simulink model "ProjectSimulink"  (R2021a)
settings: Solver=ode23  StartTime=60000  StopTime=70000  MaxStep=0.01  RelTol=1e-3
values from neighbouring files (symbols this model uses):
  Cn = Cn_cell*Np    [ProjectMatlab_Final.m]
  diesel_cap_pu = diesel_cap/Psysbase    (= 0.284375)    [ProjectMatlab_Final.m]
  EFF = 0.93    [ProjectMatlab_Final.m]
  H = 5    [ProjectMatlab_Final.m]
  k = 0.5    [ProjectMatlab_Final.m]
  k_bat = 0.5    [ProjectMatlab_Final.m]
  k_PV = 0.5    [ProjectMatlab_Final.m]
  Kii = wi^2*L/udc    (= 0.000555555555556)    [ProjectMatlab_Final.m]
  Kpi = 2*xii*wi*L/udc    (= 7.77777777778e-05)    [ProjectMatlab_Final.m]
  Ksoc = 100*(Irated*0.05)    [ProjectMatlab_Final.m]
  L = 0.005    [ProjectMatlab_Final.m]
  load_0 = 0.5    [ProjectMatlab_Final.m]
  load_0_bat = (load_0 - penetration)*Psysbase/Pgenbase    (= -0.3)    [ProjectMatlab_Final.m]
  load_0_synch = 0    [ProjectMatlab_Final.m]
  OCV_0 = interp1(SOC_LUT,OCV_LUT,SOC_0,'linear','extrap')    [ProjectMatlab_Final.m]
  OCV_LUT = Ns*OCV_LUT_cell'    [ProjectMatlab_Final.m]
  Psysbase = 320    [ProjectMatlab_Final.m]
  R = 0.03    [ProjectMatlab_Final.m]
  R_PV = 0.1    [ProjectMatlab_Final.m]
  Rb = R_cell*Ns/Np    [ProjectMatlab_Final.m]
  Rf = 0.05    [ProjectMatlab_Final.m]
  SOC_0 = 0.7    [ProjectMatlab_Final.m]
  SOC_LUT = [0.0066 0.1004 0.2004 0.3003 0.4002 0.5002 0.6001 0.7000 0.8000 0.8999 0.9998]'    [ProjectMatlab_Final.m]
  storage_p = bat_power_cap/Psysbase    (= 0.3343125)    [ProjectMatlab_Final.m]
  TCH = 0.3    [ProjectMatlab_Final.m]
  TG = 0.2    [ProjectMatlab_Final.m]
  Ub_exp = max(OCV_LUT)    [ProjectMatlab_Final.m]
  Ub_min = min(OCV_LUT)    [ProjectMatlab_Final.m]
  udc = storage_u * 1.5    (= 900)    [ProjectMatlab_Final.m]
  wbase = 2*pi*50    (= 314.159265359)    [ProjectMatlab_Final.m]
libraries: simulink x6
settings Model: Creator=bendiksherbold  LastModifiedBy=bendiksherbold
settings SolverCC: ZeroCrossAlgorithm=Adaptive
settings DataIOCC: ExternalInput=pv_data,timeseries_load  LoadExternalInput=on
settings DebuggingCC: IgnoredZcDiagnostic=none

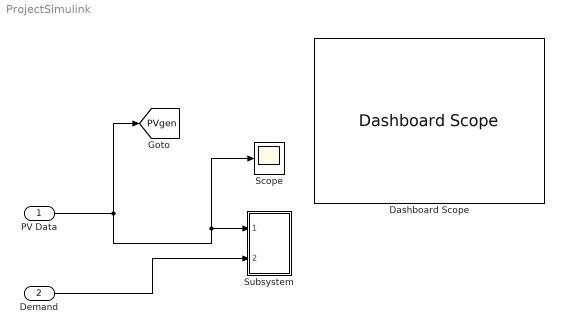
== system ProjectSimulink ==
  PV Data : Inport
  Demand : Inport  Port=2
  Dashboard Scope : DashboardScope
  Scope : Scope
  Subsystem : Subsystem
  tag scope: PVgen=global
  wires:
  PV Data/1 -> Scope/1, Subsystem/1(Renewables Input), [PVgen]
  Demand/1 -> Subsystem/2(Demand)

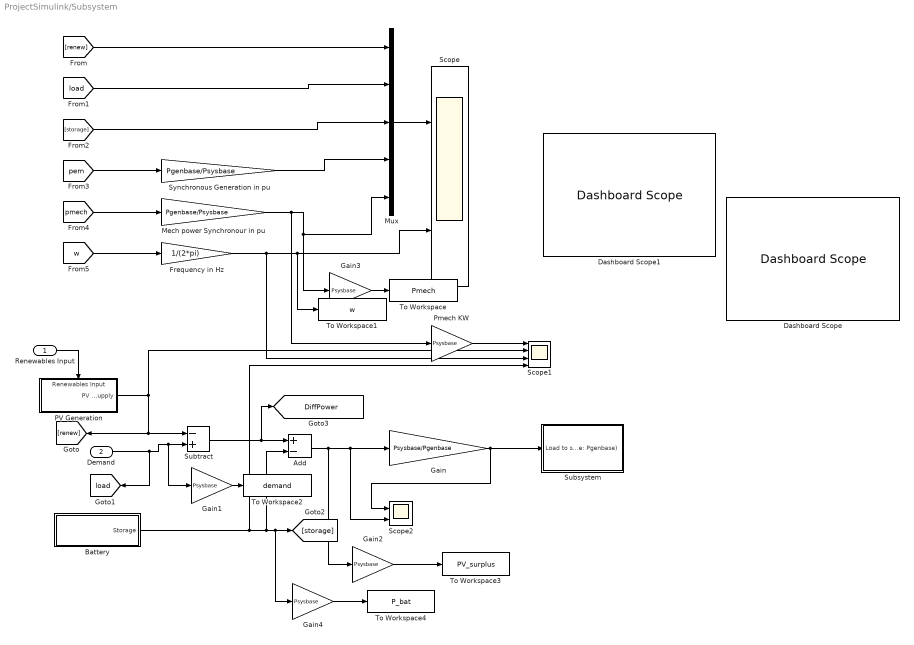
== system ProjectSimulink/Subsystem ==
  Renewables Input : Inport
  Demand : Inport  Port=2
  Add : Sum  Inputs=+-
  Battery : Subsystem
  Dashboard Scope : DashboardScope
  Dashboard Scope1 : DashboardScope
  Frequency in Hz : Gain  Gain=1/(2*pi)
  Gain : Gain  Gain=Psysbase/Pgenbase
  Gain{1..4} (4 alike) : Gain  Gain=Psysbase
  Mech power Synchronour in pu : Gain  Gain=Pgenbase/Psysbase
  Mux : Mux  Inputs=5
  PV Generation : Subsystem
      settings: PortSchema="{\"entries\":[{\"content\":{\"sides\":[{\"content\":{\"connectorIds\":[]},\"type\":\"ConnectorPlacement.EquallySpacedRectSide\",\"uuid\":\"0eea5417-339e-48e3-be8a-7ac1e3b13c5e\"},{\"content\":{\"connectorIds\":[\"Out1\"],\"side\":\"RIGHT\"},\"type\":\"ConnectorPlacement.EquallySpacedRectSide\",\"uuid\":\"a12bbc12-1de9-45f8-93a0-544242284c74\"},{\"content\":{\"connectorIds\":[\"In1\"],\"side\":\"TOP\"},\"type\":\"ConnectorPlacement.EquallySpacedRectSide\",\"uuid\":\"cdfd9bc5-7ff1-4687-a49b-7b50cbbba0d4\"}]},\"type\":\"ConnectorPlacement.EquallySpacedConnector\",\"uuid\":\"d3b80c90-fca6-417c-b380-4dfc861acc4c\"}],\"packageUris\":[\"http://schema.mathworks.com/mf0/Connector/R2020b\"],\"version\":\"1.0\"}"
  Pmech KW : Gain  Gain=Psysbase
  Scope : Scope  NumInputPorts=2
  Scope1 : Scope  NumInputPorts=4
  Scope2 : Scope  NumInputPorts=2
  Subsystem : Subsystem
  Subtract : Sum  Inputs=-+
  Synchronous Generation in pu : Gain  Gain=Pgenbase/Psysbase
  To Workspace : ToWorkspace  VariableName=Pmech  SaveFormat=Timeseries  SampleTime=-1
  To Workspace1 : ToWorkspace  VariableName=w  SaveFormat=Timeseries  SampleTime=-1
  To Workspace2 : ToWorkspace  VariableName=demand  SaveFormat=Timeseries  SampleTime=-1
  To Workspace3 : ToWorkspace  VariableName=PV_surplus  SaveFormat=Timeseries  SampleTime=-1
  To Workspace4 : ToWorkspace  VariableName=P_bat  SaveFormat=Timeseries  SampleTime=-1
  tag scope: DiffPower=global, load=global
  wires:
  [renew] -> Mux/1
  [load] -> Mux/2
  [storage] -> Mux/3
  [pem] -> Synchronous Generation in pu/1
  Synchronous Generation in pu/1 -> Mux/4
  [pmech] -> Mech power Synchronour in pu/1
  [w] -> Frequency in Hz/1
  Mux/1 -> Scope/1
  Frequency in Hz/1 -> Scope1/3, To Workspace1/1, Scope/2
  Gain/1 -> Subsystem/1(Load to synch generator (pu base: Pgenbase)), Scope2/1
  Subtract/1 -> Add/1, [DiffPower]
  Battery/1(Storage) -> Scope1/4, Add/2, Gain4/1, [storage]
  Add/1 -> Gain2/1, Scope2/2, Gain/1
  PV Generation/1(PV Power supply) -> [renew], Subtract/1, Scope1/2
  Renewables Input/1 -> PV Generation/1(Renewables Input)
  Demand/1 -> [load], Gain1/1, Subtract/2
  Gain1/1 -> To Workspace2/1
  Gain2/1 -> To Workspace3/1
  Gain3/1 -> To Workspace/1
  Mech power Synchronour in pu/1 -> Pmech KW/1, Mux/5, Gain3/1
  Pmech KW/1 -> Scope1/1
  Gain4/1 -> To Workspace4/1

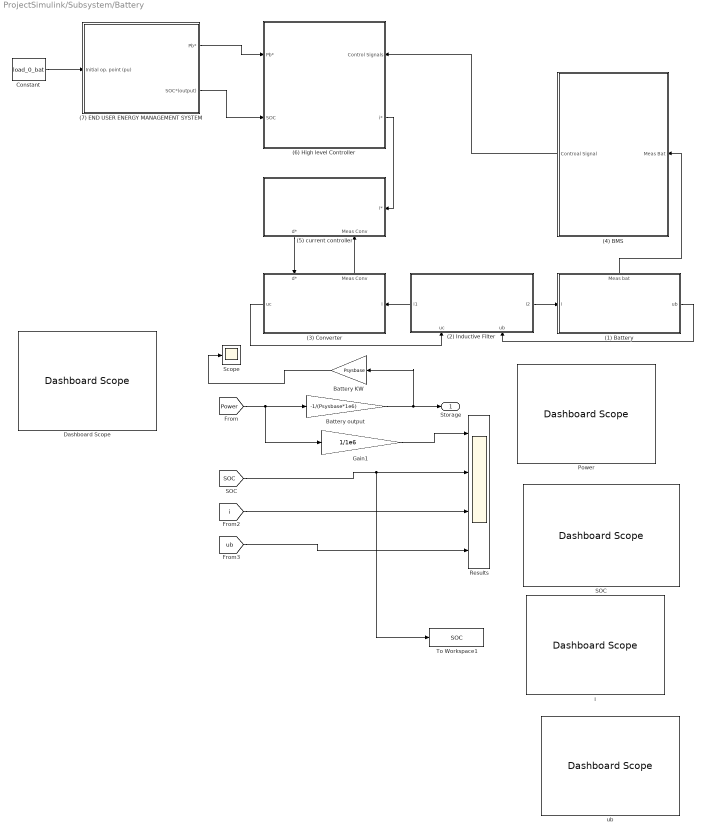
== system ProjectSimulink/Subsystem/Battery ==
  " SOC" : DashboardScope
  (1) Battery : Subsystem
      settings: PortSchema="{\"entries\":[{\"content\":{\"sides\":[{\"content\":{\"connectorIds\":[\"In1\"]},\"type\":\"ConnectorPlacement.EquallySpacedRectSide\",\"uuid\":\"e34c45c3-0268-41b7-a456-a7ff7a17db6e\"},{\"content\":{\"connectorIds\":[\"Out1\"],\"side\":\"RIGHT\"},\"type\":\"ConnectorPlacement.EquallySpacedRectSide\",\"uuid\":\"7704b9d9-7556-456b-9f5a-c4d56f80ae30\"},{\"content\":{\"connectorIds\":[\"Out2\"],\"side\":\"TOP\"},\"type\":\"ConnectorPlacement.EquallySpacedRectSide\",\"uuid\":\"0449123b-420b-4c01-93d9-a7aad71b96da\"}]},\"type\":\"ConnectorPlacement.EquallySpacedConnector\",\"uuid\":\"13f32f51-f15f-4766-88e8-e2ed957cd412\"}],\"packageUris\":[\"http://schema.mathworks.com/mf0/Connector/R2020b\"],\"version\":\"1.0\"}"
  (2) Inductive Filter : Subsystem
      settings: PortSchema="{\"entries\":[{\"content\":{\"sides\":[{\"content\":{\"connectorIds\":[\"Out2\"]},\"type\":\"ConnectorPlacement.EquallySpacedRectSide\",\"uuid\":\"c9490074-2b7b-4447-a33c-a9379d322631\"},{\"content\":{\"connectorIds\":[\"Out1\"],\"side\":\"RIGHT\"},\"type\":\"ConnectorPlacement.EquallySpacedRectSide\",\"uuid\":\"2ec79e2c-d8dd-4257-943e-016b77f5a984\"},{\"content\":{\"connectorIds\":[],\"side\":\"TOP\"},\"type\":\"ConnectorPlacement.EquallySpacedRectSide\",\"uuid\":\"d6c4e837-3256-4e0a-b933-06ad8d5ab609\"},{\"content\":{\"connectorIds\":[\"In1\",\"In2\"],\"side\":\"BOTTOM\"},\"type\":\"ConnectorPlacement.EquallySpacedRectSide\",\"uuid\":\"4075f384-4c82-404c-bba4-24b3ea83b751\"}]},\"type\":\"ConnectorPlacement.EquallySpacedConnector\",\"uuid\":\"d50deaef-6ab5-4075-8ac8-83e9d6338d4a\"}],\"packageUris\":[\"http://schema.mathworks.com/mf0/Connector/R2020b\"],\"version\":\"1.0\"}"
  (3) Converter : Subsystem
      settings: PortSchema="{\"entries\":[{\"content\":{\"sides\":[{\"content\":{\"connectorIds\":[\"Out2\"]},\"type\":\"ConnectorPlacement.EquallySpacedRectSide\",\"uuid\":\"c9490074-2b7b-4447-a33c-a9379d322631\"},{\"content\":{\"connectorIds\":[\"In2\"],\"side\":\"RIGHT\"},\"type\":\"ConnectorPlacement.EquallySpacedRectSide\",\"uuid\":\"2ec79e2c-d8dd-4257-943e-016b77f5a984\"},{\"content\":{\"connectorIds\":[\"In1\",\"Out1\"],\"side\":\"TOP\"},\"type\":\"ConnectorPlacement.EquallySpacedRectSide\",\"uuid\":\"d6c4e837-3256-4e0a-b933-06ad8d5ab609\"}]},\"type\":\"ConnectorPlacement.EquallySpacedConnector\",\"uuid\":\"d50deaef-6ab5-4075-8ac8-83e9d6338d4a\"}],\"packageUris\":[\"http://schema.mathworks.com/mf0/Connector/R2020b\"],\"version\":\"1.0\"}"
  (4) BMS : Subsystem
      settings: PortSchema="{\"entries\":[{\"content\":{\"sides\":[{\"content\":{\"connectorIds\":[\"Out1\"]},\"type\":\"ConnectorPlacement.EquallySpacedRectSide\",\"uuid\":\"7ad5997f-ae27-4a98-8ab9-418effdbae5c\"},{\"content\":{\"connectorIds\":[\"In1\"],\"side\":\"RIGHT\"},\"type\":\"ConnectorPlacement.EquallySpacedRectSide\",\"uuid\":\"c56e7a01-525e-484f-a434-88ecf8a546e8\"},{\"content\":{\"connectorIds\":[],\"side\":\"TOP\"},\"type\":\"ConnectorPlacement.EquallySpacedRectSide\",\"uuid\":\"617b0b0b-0700-4f1b-a6c2-75a7b65ee563\"},{\"content\":{\"connectorIds\":[],\"side\":\"BOTTOM\"},\"type\":\"ConnectorPlacement.EquallySpacedRectSide\",\"uuid\":\"8f108a49-84c7-4e3f-a676-05e2ecd3a647\"}]},\"type\":\"ConnectorPlacement.EquallySpacedConnector\",\"uuid\":\"a459534c-8992-4e34-9193-d09d3abfd6a6\"}],\"packageUris\":[\"http://schema.mathworks.com/mf0/Connector/R2020b\"],\"version\":\"1.0\"}"
  (5) current controller : Subsystem
      settings: PortSchema="{\"entries\":[{\"content\":{\"sides\":[{\"content\":{\"connectorIds\":[]},\"type\":\"ConnectorPlacement.EquallySpacedRectSide\",\"uuid\":\"2d354075-c17d-4344-a815-85536605997e\"},{\"content\":{\"connectorIds\":[\"In2\"],\"side\":\"RIGHT\"},\"type\":\"ConnectorPlacement.EquallySpacedRectSide\",\"uuid\":\"9e91ce6a-f1ef-4336-bc5a-278a409c018d\"},{\"content\":{\"connectorIds\":[],\"side\":\"TOP\"},\"type\":\"ConnectorPlacement.EquallySpacedRectSide\",\"uuid\":\"a4716af3-f2b8-45e2-a3c3-6e76ca82c58b\"},{\"content\":{\"connectorIds\":[\"Out1\",\"In1\"],\"side\":\"BOTTOM\"},\"type\":\"ConnectorPlacement.EquallySpacedRectSide\",\"uuid\":\"8f9d6488-9f86-4c0c-8bcc-8928f445b617\"}]},\"type\":\"ConnectorPlacement.EquallySpacedConnector\",\"uuid\":\"f4ac1926-eca6-4ae4-a6e1-7b825295d917\"}],\"packageUris\":[\"http://schema.mathworks.com/mf0/Connector/R2020b\"],\"version\":\"1.0\"}"
  (6) High level Controller : Subsystem
      settings: PortSchema="{\"entries\":[{\"content\":{\"sides\":[{\"content\":{\"connectorIds\":[\"In1\",\"In2\"]},\"type\":\"ConnectorPlacement.EquallySpacedRectSide\",\"uuid\":\"f1980330-cce1-4eae-bd21-bb2edf6a6354\"},{\"content\":{\"connectorIds\":[\"In3\",\"Out1\"],\"side\":\"RIGHT\"},\"type\":\"ConnectorPlacement.EquallySpacedRectSide\",\"uuid\":\"5b150bd5-b030-427f-a8ee-89c6d0847365\"},{\"content\":{\"connectorIds\":[],\"side\":\"TOP\"},\"type\":\"ConnectorPlacement.EquallySpacedRectSide\",\"uuid\":\"ea0f71d8-017f-4572-8166-56d940581349\"}]},\"type\":\"ConnectorPlacement.EquallySpacedConnector\",\"uuid\":\"37bf4f98-7efc-4bdf-9457-78864a4c59b2\"}],\"packageUris\":[\"http://schema.mathworks.com/mf0/Connector/R2020b\"],\"version\":\"1.0\"}"
  (7) END USER ENERGY MANAGEMENT SYSTEM : Subsystem
  Battery KW : Gain  Gain=Psysbase
  Battery output : Gain  Gain=-1/(Psysbase*1e6)
  Constant : Constant  Value=load_0_bat
  Dashboard Scope : DashboardScope
  Gain1 : Gain  Gain=1/1e6
  Power : DashboardScope
  Results : Scope  NumInputPorts=4
  Scope : Scope
  To Workspace1 : ToWorkspace  VariableName=SOC  SaveFormat=Timeseries  SampleTime=-1
      settings: Save2DSignal=2-D array (concatenate along first dimension)
  i : DashboardScope
  ub : DashboardScope
  Storage : Outport
  wires:
  (1) Battery/1(ub) -> (2) Inductive Filter/2(ub)
  (2) Inductive Filter/1(i2) -> (1) Battery/1(i)
  (3) Converter/2(uc) -> (2) Inductive Filter/1(uc)
  (2) Inductive Filter/2(i1) -> (3) Converter/2(i)
  (1) Battery/2(Meas bat) -> (4) BMS/1(Meas Bat)
  (5) current controller/1(d*) -> (3) Converter/1(d*)
  (3) Converter/1(Meas Conv) -> (5) current controller/1(Meas Conv)
  [Power] -> Gain1/1, Battery output/1
  Battery output/1 -> Battery KW/1, Storage/1
  [ub] -> Results/4
  [i] -> Results/3
  [SOC] -> To Workspace1/1, Results/2
  Gain1/1 -> Results/1
  (7) END USER ENERGY MANAGEMENT SYSTEM/1(Pb*) -> (6) High level Controller/1(Pb*)
  (7) END USER ENERGY MANAGEMENT SYSTEM/2(SOC*(output)) -> (6) High level Controller/2(SOC)
  (4) BMS/1(Controal Signal) -> (6) High level Controller/3(Control Signals)
  (6) High level Controller/1(i*) -> (5) current controller/2(i*)
  Constant/1 -> (7) END USER ENERGY MANAGEMENT SYSTEM/1(Initial op. point (pu))
  Battery KW/1 -> Scope/1

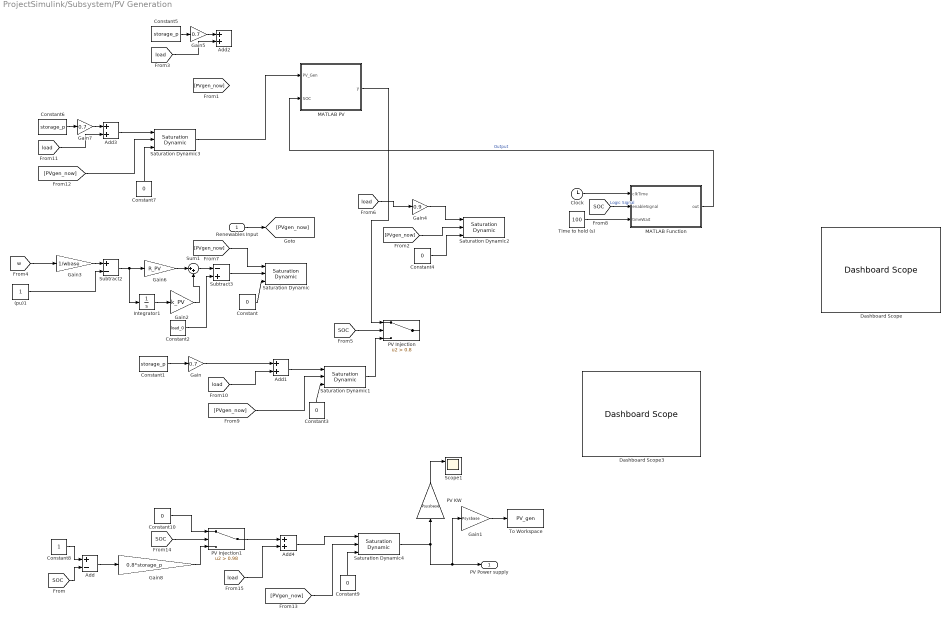
== system ProjectSimulink/Subsystem/PV Generation ==
  Renewables Input : Inport
  (pu)1 : Constant
  Add : Sum  Inputs=+-
  Add{1..4} (4 alike) : Sum
  Clock : Clock
  Constant{,3..4,7,9..10} (6 alike) : Constant  Value=0
  Constant1 : Constant  Value=storage_p
  Constant2 : Constant  Value=load_0
  Constant5 : Constant  Value=storage_p
  Constant6 : Constant  Value=storage_p
  Constant8 : Constant
  Dashboard Scope : DashboardScope
  Dashboard Scope3 : DashboardScope
  Gain : Gain  Gain=0.7
  Gain1 : Gain  Gain=Psysbase
  Gain2 : Gain  Gain=k_PV
  Gain3 : Gain  Gain=1/wbase
  Gain4 : Gain  Gain=0.9
  Gain5 : Gain  Gain=0.7
  Gain6 : Gain  Gain=R_PV
  Gain7 : Gain  Gain=0.7
  Gain8 : Gain  Gain=0.8*storage_p
  Integrator1 : Integrator
  MATLAB Function : MATLAB Function  TreatAsAtomicUnit=on
  MATLAB PV : MATLAB Function  TreatAsAtomicUnit=on
  PV Injection : Switch  Criteria=u2 > Threshold  Threshold=0.8
  PV Injection1 : Switch  Criteria=u2 > Threshold  Threshold=0.98
  PV KW : Gain  Gain=Psysbase
  Saturation Dynamic{,1..4} (5 alike) : simulink/Discontinuities/Saturation Dynamic  OutMin=[]  OutMax=[]  OutDataTypeStr=Inherit: Same as second input  OutDataType=fixdt(1, 16)  OutScaling=2^-10  DoSatur=off
  Scope1 : Scope  NumInputPorts=2
  Subtract2 : Sum  Inputs=+-
  Subtract3 : Sum  Inputs=-+
  Sum1 : Sum  Inputs=|++
  Time to hold (s) : Constant  Value=100
  To Workspace : ToWorkspace  VariableName=PV_gen  SaveFormat=Timeseries  SampleTime=-1
  PV Power supply : Outport
  wires:
  Constant/1 -> Saturation Dynamic/3
  Constant2/1 -> Subtract3/2
  Gain3/1 -> Subtract2/1
  (pu)1/1 -> Subtract2/2
  Subtract2/1 -> Integrator1/1, Gain6/1
  Gain2/1 -> Sum1/2
  Gain6/1 -> Sum1/1
  [w] -> Gain3/1
  Sum1/1 -> Subtract3/1
  Integrator1/1 -> Gain2/1
  Subtract3/1 -> Saturation Dynamic/2
  Renewables Input/1 -> [PVgen_now]
  [PVgen_now] -> Saturation Dynamic/1
  Saturation Dynamic1/1 -> PV Injection/3
  Constant3/1 -> Saturation Dynamic1/3
  Constant1/1 -> Gain/1
  [load] -> Add1/2
  Add1/1 -> Saturation Dynamic1/1
  [PVgen_now] -> Saturation Dynamic1/2
  Gain1/1 -> To Workspace/1
  PV KW/1 -> Scope1/1
  [PVgen_now] -> Saturation Dynamic2/2
  Constant4/1 -> Saturation Dynamic2/3
  Gain/1 -> Add1/1
  [load] -> Gain4/1
  Gain4/1 -> Saturation Dynamic2/1
  [SOC] -> MATLAB Function/2(enableSignal)  "Logic Signal"
  Time to hold (s)/1 -> MATLAB Function/3(timeWait)
  Clock/1 -> MATLAB Function/1(clkTime)
  [SOC] -> PV Injection/2
  MATLAB Function/1(out) -> MATLAB PV/2(SOC)  "Output"
  MATLAB PV/1(y) -> PV Injection/1
  Gain5/1 -> Add2/1
  Constant5/1 -> Gain5/1
  [load] -> Add2/2
  Gain7/1 -> Add3/1
  [PVgen_now] -> Saturation Dynamic3/2
  Constant6/1 -> Gain7/1
  Constant7/1 -> Saturation Dynamic3/3
  [load] -> Add3/2
  Add3/1 -> Saturation Dynamic3/1
  Saturation Dynamic3/1 -> MATLAB PV/1(PV_Gen)
  Constant8/1 -> Add/1
  [SOC] -> Add/2
  Add/1 -> Gain8/1
  [PVgen_now] -> Saturation Dynamic4/2
  Constant9/1 -> Saturation Dynamic4/3
  [SOC] -> PV Injection1/2
  Constant10/1 -> PV Injection1/1
  [load] -> Add4/2
  Add4/1 -> Saturation Dynamic4/1
  Gain8/1 -> PV Injection1/3
  PV Injection1/1 -> Add4/1
  Saturation Dynamic4/1 -> PV KW/1, Gain1/1, PV Power supply/1

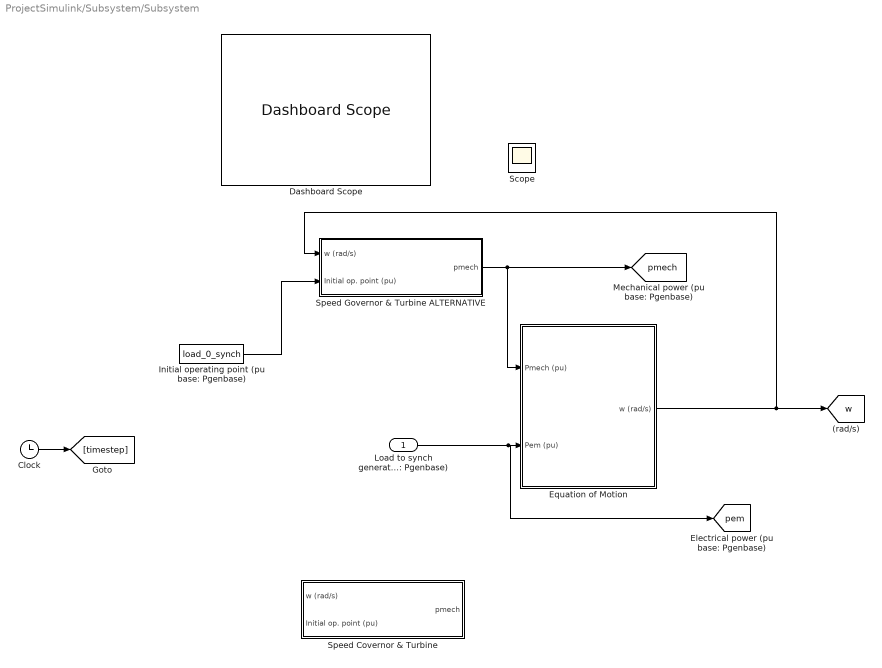
== system ProjectSimulink/Subsystem/Subsystem ==
  Load to synch generator (pu base: Pgenbase) : Inport
  Clock : Clock
  Dashboard Scope : DashboardScope
  Equation of Motion : Subsystem
  Initial operating point (pu base: Pgenbase) : Constant  Value=load_0_synch
  Scope : Scope
  Speed Covernor & Turbine : Subsystem
  Speed Governor & Turbine ALTERNATIVE : Subsystem
  tag scope: pem=global, pmech=global, w=global
  wires:
  Load to synch generator (pu base: Pgenbase)/1 -> [pem], Equation of Motion/2(Pem (pu))
  Equation of Motion/1(w (rad/s)) -> Speed Governor & Turbine ALTERNATIVE/1(w (rad/s)), [w]
  Clock/1 -> [timestep]
  Speed Governor & Turbine ALTERNATIVE/1(pmech) -> Equation of Motion/1(Pmech (pu)), [pmech]
  Initial operating point (pu base: Pgenbase)/1 -> Speed Governor & Turbine ALTERNATIVE/2(Initial op. point (pu))

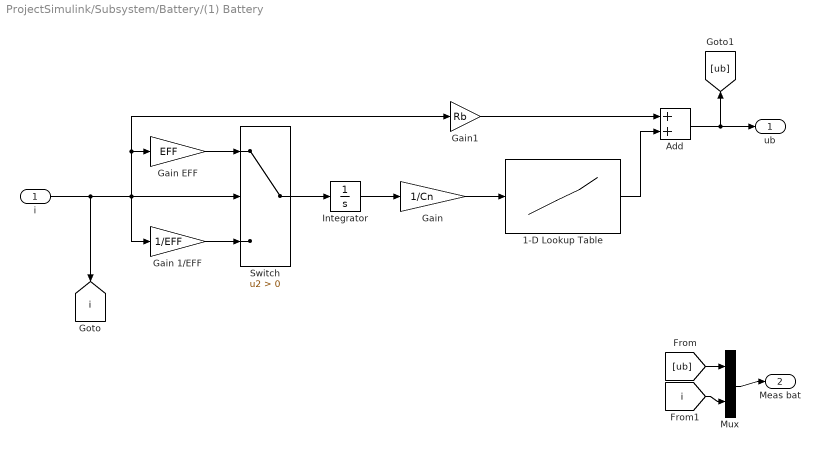
== system ProjectSimulink/Subsystem/Battery/(1) Battery ==
  i : Inport
  1-D Lookup Table : Lookup_n-D  NumberOfTableDimensions=1  BreakpointsForDimension1=SOC_LUT  Table=OCV_LUT  InternalRulePriority=Speed  RndMeth=Simplest  InputSameDT=on
  Add : Sum
  Gain : Gain  Gain=1/Cn
  Gain 1/EFF : Gain  Gain=1/EFF
  Gain EFF : Gain  Gain=EFF
  Gain1 : Gain  Gain=Rb
  Integrator : Integrator  InitialCondition=SOC_0*Cn
  Mux : Mux  Inputs=2
  Switch : Switch  Criteria=u2 > Threshold
  ub : Outport
  Meas bat : Outport  Port=2
  tag scope: i=global
  wires:
  i/1 -> [i], Gain 1/EFF/1, Gain1/1, Gain EFF/1, Switch/2
  Switch/1 -> Integrator/1
  Integrator/1 -> Gain/1
  Gain/1 -> 1-D Lookup Table/1
  Add/1 -> [ub], ub/1
  Gain EFF/1 -> Switch/1
  Gain 1/EFF/1 -> Switch/3
  Gain1/1 -> Add/1
  1-D Lookup Table/1 -> Add/2
  [i] -> Mux/2
  [ub] -> Mux/1
  Mux/1 -> Meas bat/1

== system ProjectSimulink/Subsystem/Battery/(2) Inductive Filter ==
  uc : Inport
  ub : Inport  Port=2
  Add : Sum  Inputs=+-
  Gain : Gain  Gain=1/L
  Integrator : Integrator
  i2 : Outport
  i1 : Outport  Port=2
  wires:
  uc/1 -> Add/1
  ub/1 -> Add/2
  Add/1 -> Gain/1
  Gain/1 -> Integrator/1
  Integrator/1 -> i2/1, i1/1

== system ProjectSimulink/Subsystem/Battery/(3) Converter ==
  d* : Inport
  i : Inport  Port=2
  Gain : Gain  Gain=udc
  Product : Product
  Meas Conv : Outport
  uc : Outport  Port=2
  tag scope: Power=global
  wires:
  d*/1 -> Gain/1
  Gain/1 -> Product/1, uc/1
  i/1 -> Product/2, Meas Conv/1
  Product/1 -> [Power]

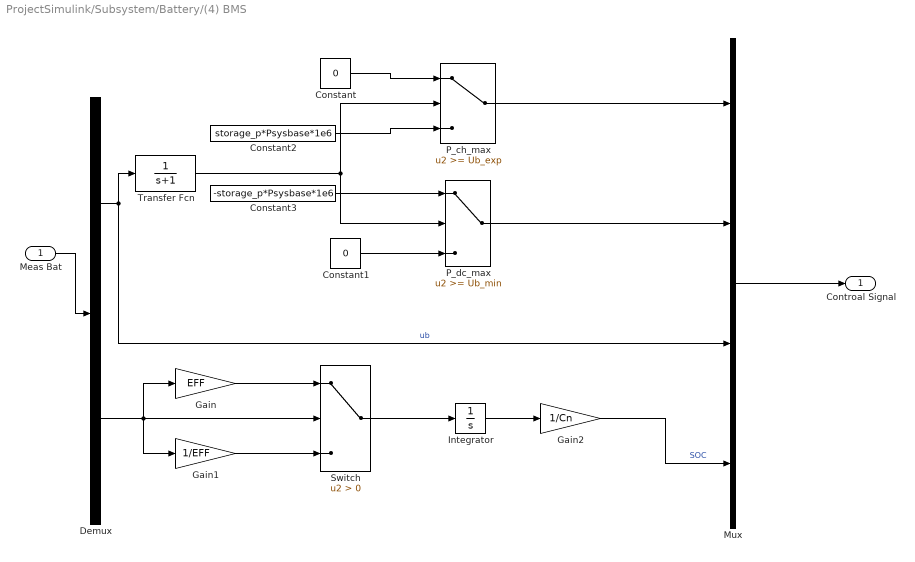
== system ProjectSimulink/Subsystem/Battery/(4) BMS ==
  Meas Bat : Inport
  Constant : Constant  Value=0
  Constant1 : Constant  Value=0
  Constant2 : Constant  Value=storage_p*Psysbase*1e6
  Constant3 : Constant  Value=-storage_p*Psysbase*1e6
  Demux : Demux  Outputs=2
  Gain : Gain  Gain=EFF
  Gain1 : Gain  Gain=1/EFF
  Gain2 : Gain  Gain=1/Cn
  Integrator : Integrator  InitialCondition=SOC_0*Cn
  Mux : Mux
  P_ch_max : Switch  Threshold=Ub_exp  ZeroCross=off
  P_dc_max : Switch  Threshold=Ub_min  ZeroCross=off
  Switch : Switch  Criteria=u2 > Threshold
  Transfer Fcn : TransferFcn  Denominator=[1 1]
  Controal Signal : Outport
  wires:
  Meas Bat/1 -> Demux/1
  Demux/1 -> Transfer Fcn/1, Mux/3  "ub"
  Transfer Fcn/1 -> P_ch_max/2, P_dc_max/2
  Constant/1 -> P_ch_max/1
  Constant1/1 -> P_dc_max/3
  Constant2/1 -> P_ch_max/3
  Constant3/1 -> P_dc_max/1
  Demux/2 -> Gain1/1, Gain/1, Switch/2
  Gain1/1 -> Switch/3
  Gain/1 -> Switch/1
  Switch/1 -> Integrator/1
  Integrator/1 -> Gain2/1
  Gain2/1 -> Mux/4  "SOC"
  P_dc_max/1 -> Mux/2
  P_ch_max/1 -> Mux/1
  Mux/1 -> Controal Signal/1

== system ProjectSimulink/Subsystem/Battery/(5) current controller ==
  Meas Conv : Inport
  i* : Inport  Port=2
  Add : Sum  Inputs=+-
  PI : Subsystem
  d* : Outport
  wires:
  i*/1 -> Add/1
  Meas Conv/1 -> Add/2
  Add/1 -> PI/1(ln)
  PI/1(d*) -> d*/1

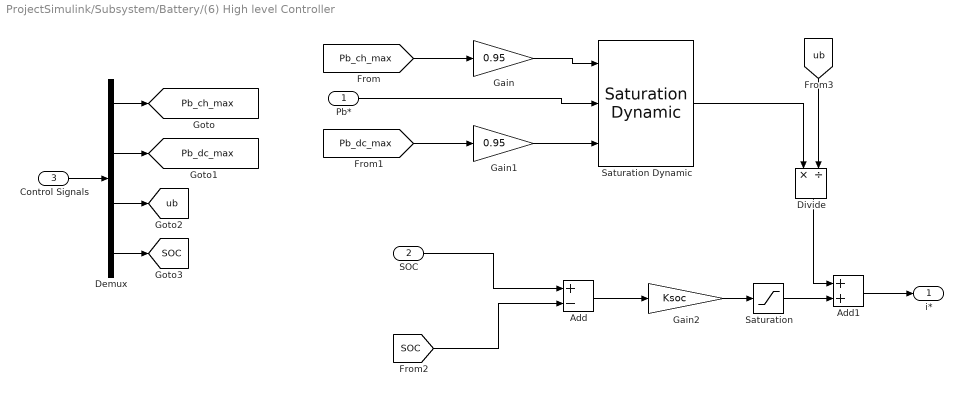
== system ProjectSimulink/Subsystem/Battery/(6) High level Controller ==
  Pb* : Inport
  SOC : Inport  Port=2
  Control Signals : Inport  Port=3
  Add : Sum  Inputs=+-
  Add1 : Sum
  Demux : Demux
  Divide : Product  Inputs=*/
  Gain : Gain  Gain=0.95
  Gain1 : Gain  Gain=0.95
  Gain2 : Gain  Gain=Ksoc
  Saturation : Saturate
  Saturation Dynamic : simulink/Discontinuities/Saturation Dynamic  OutMin=[]  OutMax=[]  OutDataTypeStr=Inherit: Same as second input  OutDataType=fixdt(1, 16)  OutScaling=2^-10  DoSatur=off
  i* : Outport
  tag scope: Pb_ch_max=global, Pb_dc_max=global, SOC=global, ub=global
  wires:
  [Pb_ch_max] -> Gain/1
  [Pb_dc_max] -> Gain1/1
  Pb*/1 -> Saturation Dynamic/2
  Gain/1 -> Saturation Dynamic/1
  Gain1/1 -> Saturation Dynamic/3
  SOC/1 -> Add/1
  [SOC] -> Add/2
  Add/1 -> Gain2/1
  Gain2/1 -> Saturation/1
  Saturation/1 -> Add1/2
  Saturation Dynamic/1 -> Divide/1
  [ub] -> Divide/2
  Divide/1 -> Add1/1
  Add1/1 -> i*/1
  Control Signals/1 -> Demux/1
  Demux/1 -> [Pb_ch_max]
  Demux/2 -> [Pb_dc_max]
  Demux/3 -> [ub]
  Demux/4 -> [SOC]

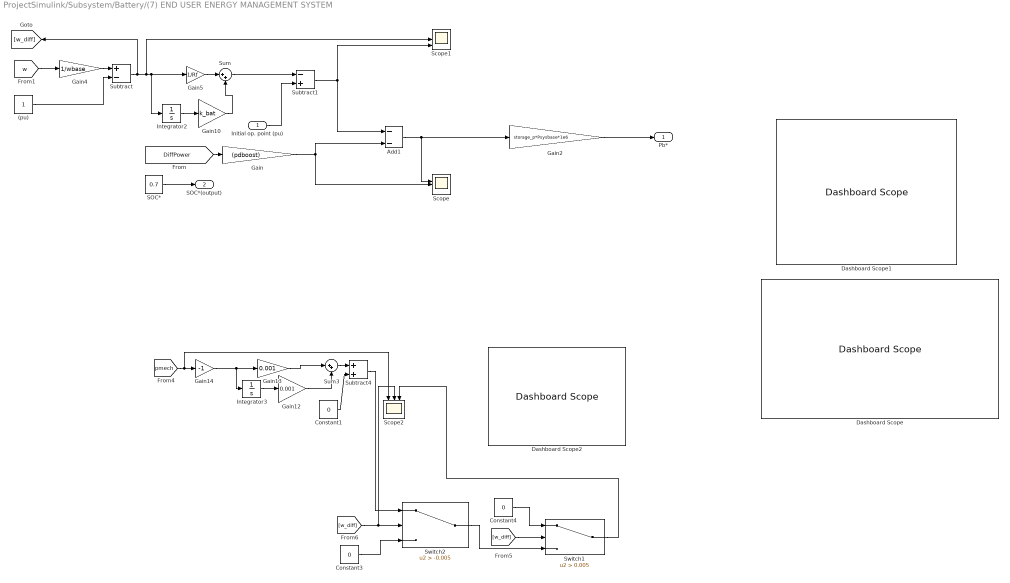
== system ProjectSimulink/Subsystem/Battery/(7) END USER ENERGY MANAGEMENT SYSTEM ==
  Initial op. point (pu) : Inport
  (pu) : Constant
  Add1 : Sum  Inputs=--
  Constant1 : Constant  Value=0
  Constant3 : Constant  Value=0
  Constant4 : Constant  Value=0
  Dashboard Scope : DashboardScope
  Dashboard Scope1 : DashboardScope
  Dashboard Scope2 : DashboardScope
  Gain : Gain  Gain=(pdboost)
  Gain10 : Gain  Gain=k_bat
  Gain12 : Gain  Gain=0.001
  Gain13 : Gain  Gain=0.001
  Gain14 : Gain  Gain=-1
  Gain2 : Gain  Gain=storage_p*Psysbase*1e6
  Gain4 : Gain  Gain=1/wbase
  Gain5 : Gain  Gain=1/Rf
  Integrator2 : Integrator
  Integrator3 : Integrator
  SOC* : Constant  Value=0.7
  Scope : Scope  NumInputPorts=5
  Scope1 : Scope  NumInputPorts=3
  Scope2 : Scope  NumInputPorts=3
  Subtract : Sum  Inputs=+-
  Subtract1 : Sum  Inputs=-+
  Subtract4 : Sum
  Sum : Sum  Inputs=|++
  Sum3 : Sum  Inputs=|++
  Switch1 : Switch  Criteria=u2 > Threshold  Threshold=0.005
  Switch2 : Switch  Criteria=u2 > Threshold  Threshold=-0.005
  Pb* : Outport
  SOC*(output) : Outport  Port=2
  wires:
  [DiffPower] -> Gain/1
  Gain2/1 -> Pb*/1
  SOC*/1 -> SOC*(output)/1
  Gain/1 -> Scope/3, Add1/2
  Gain4/1 -> Subtract/1
  Gain5/1 -> Sum/1
  (pu)/1 -> Subtract/2
  Subtract/1 -> [w_diff], Scope1/2, Integrator2/1, Gain5/1
  Initial op. point (pu)/1 -> Subtract1/2
  Gain10/1 -> Sum/2
  Integrator2/1 -> Gain10/1
  [w] -> Gain4/1
  Sum/1 -> Subtract1/1
  Subtract1/1 -> Scope1/3, Add1/1
  [pmech] -> Scope2/1, Gain14/1
  Integrator3/1 -> Gain12/1
  Gain13/1 -> Sum3/1
  Gain12/1 -> Sum3/2
  Gain14/1 -> Integrator3/1, Gain13/1
  Sum3/1 -> Subtract4/1
  Constant1/1 -> Subtract4/2
  Constant3/1 -> Switch2/3
  [w_diff] -> Switch1/2
  [w_diff] -> Scope2/2, Switch2/2
  Subtract4/1 -> Switch2/1
  Switch1/1 -> Scope2/3
  Constant4/1 -> Switch1/1
  Switch2/1 -> Switch1/3
  Add1/1 -> Gain2/1, Scope/2

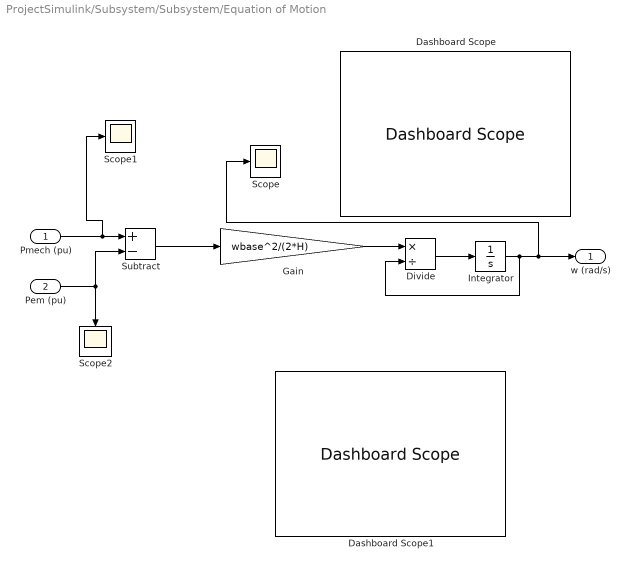
== system ProjectSimulink/Subsystem/Subsystem/Equation of Motion ==
  Pmech (pu) : Inport
  Pem (pu) : Inport  Port=2
  Dashboard Scope : DashboardScope
  Dashboard Scope1 : DashboardScope
  Divide : Product  Inputs=*/
  Gain : Gain  Gain=wbase^2/(2*H)
  Integrator : Integrator  InitialCondition=wbase
  Scope : Scope
  Scope1 : Scope
  Scope2 : Scope
  Subtract : Sum  Inputs=+-
  w (rad/s) : Outport
  wires:
  Divide/1 -> Integrator/1
  Gain/1 -> Divide/1
  Pem (pu)/1 -> Scope2/1, Subtract/2
  Pmech (pu)/1 -> Subtract/1, Scope1/1
  Integrator/1 -> Scope/1, w (rad/s)/1, Divide/2
  Subtract/1 -> Gain/1

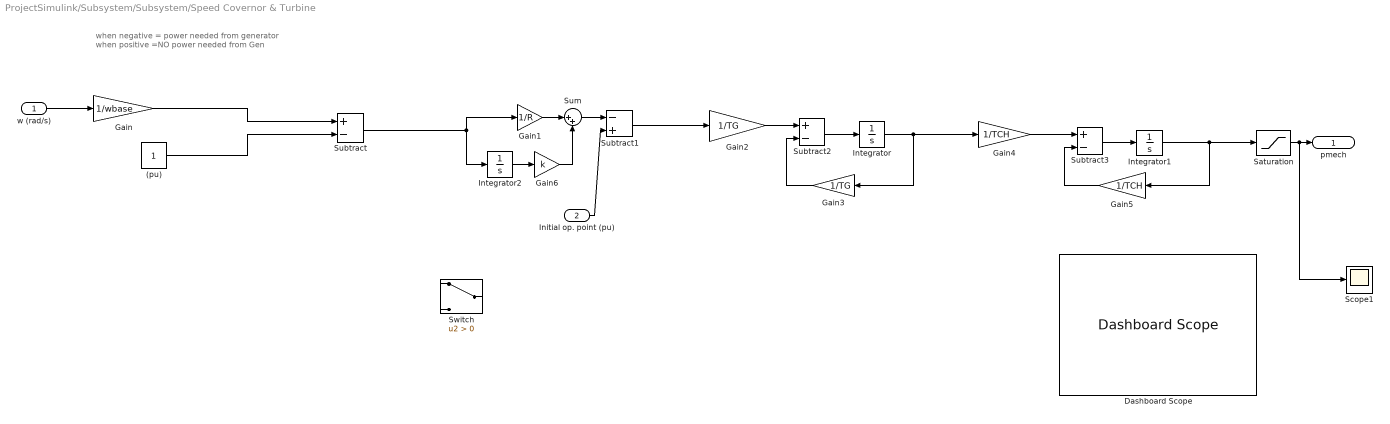
== system ProjectSimulink/Subsystem/Subsystem/Speed Covernor & Turbine ==
  note: when negative = power needed from generator
      |
      | when positive =NO power needed from Gen
  w (rad/s) : Inport
  Initial op. point (pu) : Inport  Port=2
  (pu) : Constant
  Dashboard Scope : DashboardScope
  Gain : Gain  Gain=1/wbase
  Gain1 : Gain  Gain=1/R
  Gain2 : Gain  Gain=1/TG
  Gain3 : Gain  Gain=1/TG
  Gain4 : Gain  Gain=1/TCH
  Gain5 : Gain  Gain=1/TCH
  Gain6 : Gain  Gain=k
  Integrator : Integrator  InitialCondition=load_0_synch
  Integrator1 : Integrator  InitialCondition=load_0_synch
  Integrator2 : Integrator
  Saturation : Saturate  UpperLimit=diesel_cap_pu  LowerLimit=0
  Scope1 : Scope
  Subtract : Sum  Inputs=+-
  Subtract1 : Sum  Inputs=-+
  Subtract2 : Sum  Inputs=+-
  Subtract3 : Sum  Inputs=+-
  Sum : Sum  Inputs=|++
  Switch : Switch  Criteria=u2 > Threshold
  pmech : Outport
  wires:
  Subtract1/1 -> Gain2/1
  Subtract2/1 -> Integrator/1
  Gain3/1 -> Subtract2/2
  Subtract3/1 -> Integrator1/1
  Gain4/1 -> Subtract3/1
  Integrator/1 -> Gain4/1, Gain3/1
  Gain5/1 -> Subtract3/2
  Gain2/1 -> Subtract2/1
  Initial op. point (pu)/1 -> Subtract1/2
  w (rad/s)/1 -> Gain/1
  Integrator2/1 -> Gain6/1
  Gain1/1 -> Sum/1
  Sum/1 -> Subtract1/1
  Gain6/1 -> Sum/2
  Integrator1/1 -> Saturation/1, Gain5/1
  Gain/1 -> Subtract/1
  (pu)/1 -> Subtract/2
  Subtract/1 -> Gain1/1, Integrator2/1
  Saturation/1 -> Scope1/1, pmech/1

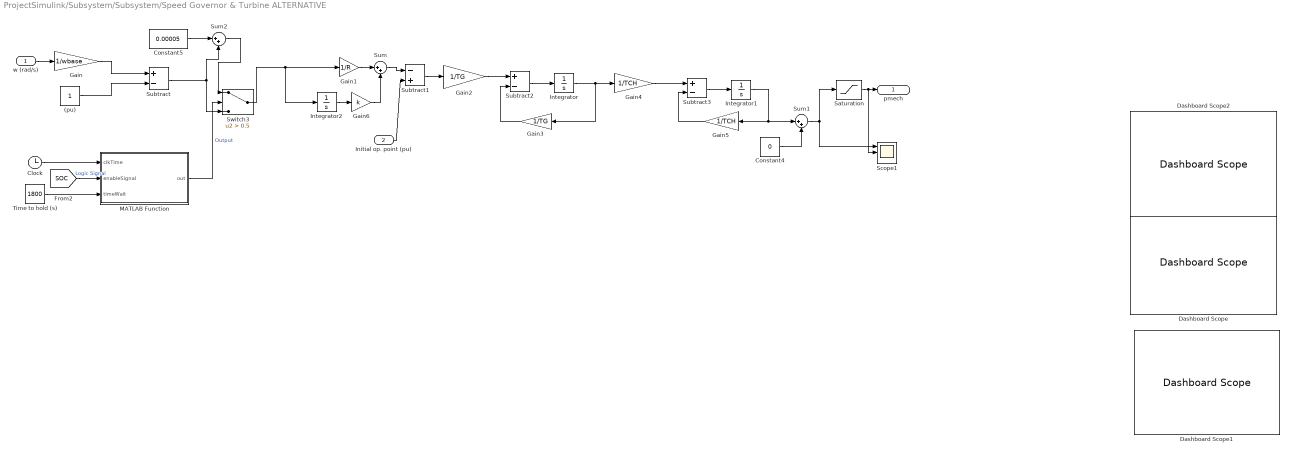
== system ProjectSimulink/Subsystem/Subsystem/Speed Governor & Turbine ALTERNATIVE ==
  w (rad/s) : Inport
  Initial op. point (pu) : Inport  Port=2
  (pu) : Constant
  Clock : Clock
  Constant4 : Constant  Value=0
  Constant5 : Constant  Value=0.00005
  Dashboard Scope : DashboardScope
  Dashboard Scope1 : DashboardScope
  Dashboard Scope2 : DashboardScope
  Gain : Gain  Gain=1/wbase
  Gain1 : Gain  Gain=1/R
  Gain2 : Gain  Gain=1/TG
  Gain3 : Gain  Gain=1/TG
  Gain4 : Gain  Gain=1/TCH
  Gain5 : Gain  Gain=1/TCH
  Gain6 : Gain  Gain=k
  Integrator : Integrator  InitialCondition=load_0_synch
  Integrator1 : Integrator  InitialCondition=load_0_synch
  Integrator2 : Integrator
  MATLAB Function : MATLAB Function  TreatAsAtomicUnit=on
  Saturation : Saturate  UpperLimit=diesel_cap_pu  LowerLimit=0
  Scope1 : Scope  NumInputPorts=3
  Subtract : Sum  Inputs=+-
  Subtract1 : Sum  Inputs=-+
  Subtract2 : Sum  Inputs=+-
  Subtract3 : Sum  Inputs=+-
  Sum : Sum  Inputs=|++
  Sum1 : Sum  Inputs=|++
  Sum2 : Sum  Inputs=|++
  Switch3 : Switch  Criteria=u2 > Threshold  Threshold=0.5
  Time to hold (s) : Constant  Value=1800
  pmech : Outport
  wires:
  Subtract1/1 -> Gain2/1
  Subtract2/1 -> Integrator/1
  Gain3/1 -> Subtract2/2
  Subtract3/1 -> Integrator1/1
  Gain4/1 -> Subtract3/1
  Integrator/1 -> Gain4/1, Gain3/1
  Gain5/1 -> Subtract3/2
  Gain2/1 -> Subtract2/1
  Initial op. point (pu)/1 -> Subtract1/2
  w (rad/s)/1 -> Gain/1
  Integrator2/1 -> Gain6/1
  Gain1/1 -> Sum/1
  Sum/1 -> Subtract1/1
  Gain6/1 -> Sum/2
  Integrator1/1 -> Sum1/1, Gain5/1
  Gain/1 -> Subtract/1
  (pu)/1 -> Subtract/2
  Saturation/1 -> Scope1/2, pmech/1
  Sum1/1 -> Saturation/1, Scope1/1
  Constant4/1 -> Sum1/2
  Clock/1 -> MATLAB Function/1(clkTime)
  [SOC] -> MATLAB Function/2(enableSignal)  "Logic Signal"
  Time to hold (s)/1 -> MATLAB Function/3(timeWait)
  MATLAB Function/1(out) -> Switch3/2  "Output"
  Subtract/1 -> Sum2/2, Switch3/3
  Switch3/1 -> Integrator2/1, Gain1/1
  Constant5/1 -> Sum2/1
  Sum2/1 -> Switch3/1

== system ProjectSimulink/Subsystem/Battery/(5) current controller/PI ==
  ln : Inport
  Add : Sum
  Gain : Gain  Gain=Kpi
  Gain1 : Gain  Gain=Kii
  Integrator : Integrator  InitialCondition=OCV_0/udc
  d* : Outport
  wires:
  ln/1 -> Gain1/1, Gain/1
  Gain/1 -> Add/1
  Add/1 -> d*/1
  Gain1/1 -> Integrator/1
  Integrator/1 -> Add/2

== matlab function ProjectSimulink/Subsystem/Subsystem/Speed Governor & Turbine ALTERNATIVE/MATLAB Function ==
  settings: updateMethod=DISCRETE
  data: clkTime input; out output; enableSignal input; timeWait input
function out = fcn(clkTime,enableSignal,timeWait)
%#codegen

% Declare persistent variables that 
persistent timeStart;
persistent preValue;

% Initialize these variables during the first time step
if isempty(preValue)
    timeStart = 0;
    preValue = enableSignal;
end

% If the wait time passes and the block is currently triggered, disabled output
if clkTime - timeStart > timeWait
    % Special condition: If we are still enabled, remain enabled. This
    % logic ensure that we remain enabled rather than turn off and
    % immediatly back on
    out = enableSignal;
    preValue = enableSignal;
    timeStart = clkTime;

else
    out = preValue;
end

== matlab function ProjectSimulink/Subsystem/PV Generation/MATLAB PV ==
  data: PV_Gen input; y output; SOC input
function y = fcn_PV( PV_Gen, SOC)

Gen = 0;

if SOC <= 0.82
   Gen = 0.8*PV_Gen; 
end
if (SOC <= 0.85) && (SOC > 0.82)
    Gen = 0.6*PV_Gen; 
end
if (SOC <= 0.9) && (SOC > 0.85)
    Gen = 0.4*PV_Gen; 
end
if (SOC <=0.95) && (SOC > 0.9) 
    Gen = 0.2*PV_Gen; 
end
if (SOC >0.95)
    Gen = 0.1*PV_Gen; 
end

y = Gen;

== matlab function ProjectSimulink/Subsystem/PV Generation/MATLAB Function ==
  settings: updateMethod=DISCRETE
  data: clkTime input; out output; enableSignal input; timeWait input
function out = fcn(clkTime,enableSignal,timeWait)
%#codegen

% Declare persistent variables that 
persistent timeStart;
persistent preValue;

% Initialize these variables during the first time step
if isempty(preValue)
    timeStart = 0;
    preValue = enableSignal;
end

% If the wait time passes and the block is currently triggered, disabled output
if clkTime - timeStart > timeWait
    % Special condition: If we are still enabled, remain enabled. This
    % logic ensure that we remain enabled rather than turn off and
    % immediatly back on
    out = enableSignal;
    preValue = enableSignal;
    timeStart = clkTime;

else
    out = preValue;
end
